simulink model "SimpleMessagesModel"  (R2019b)
settings: Solver=VariableStepAuto  StartTime=0.0  StopTime=10.0  RelTol=1e-3
libraries: simulink x1
settings Model: Creator=The MathWorks, Inc.  LastModifiedBy=bhisma

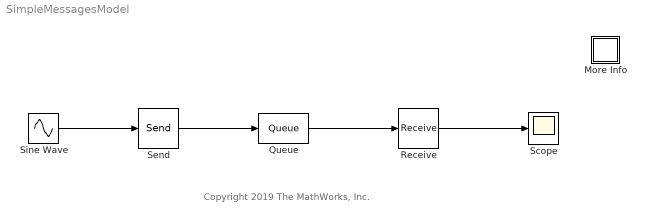
== system SimpleMessagesModel ==
  note: Copyright 2019 The MathWorks, Inc.
  More Info : Subsystem
      settings: OpenFcn=showExample('simulink/ModelMessageBasedCommunicationFrameworkExample')
      mask Display: disp('?')
  Queue : Queue  InputPortMessageModes=m  OutputPortMessageModes=m  OverwriteOldest=on  Capacity=16  QueueType=LIFO
  Receive : Receive  InputPortMessageModes=m  UseInternalQueue=off  QueueOverwriting=on  QueueLength=1  QueueType=LIFO  SampleTime=0.1
  Scope : Scope
  Send : Send  OutputPortMessageModes=m
  Sine Wave : Sin  SampleTime=0.1
  wires:
  Sine Wave/1 -> Send/1
  Send/1 -> Queue/1
  Queue/1 -> Receive/1
  Receive/1 -> Scope/1

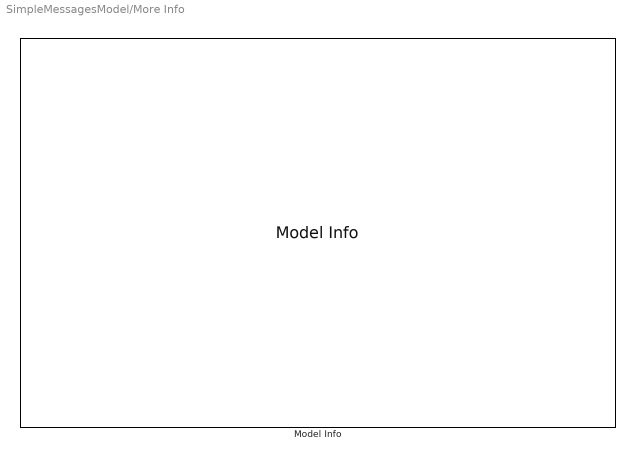
== system SimpleMessagesModel/More Info ==
  Model Info : simulink/Model-Wide Utilities/Model Info  Frame=on  DisplayStringWithTags=|  HorizontalTextAlignment=Left  LeftAlignmentValue=0.02
      | Model Description:
      | -------------------
      | This example shows how to use the Message Delay block to model a variable
      | speed conveyor belt between two airport terminals. The passengers step on
      | the conveyor belt following a Poisson distribution. Since passengers are
      | discrete entities, they are naturally modeled by Simulink(R) messages,
      | which are created by the Entity Generator block. When a passenger, i.e.,
      | a Simulink(R) message, is sent to the Message Delay block, the block
      | will hold it until it arrives at the other end of the conveyor belt. The
      | length of the delay time is automatically calculated by Simulink(R) based
      | on the ETA (estimated time of arrival), which is calculated by the
      | Stateflow(R) Chart. The operation of the conveyor belt depends on the
      | load and its transfer characteristics.
